simulink model "lab10_2"  (R2016a)
settings: Solver=VariableStepAuto  StartTime=0.0  StopTime=10.0  RelTol=1e-3
libraries: dsparch4 x1, dspsrcs4 x1
settings Model: Creator=Student  LastModifiedBy=Student

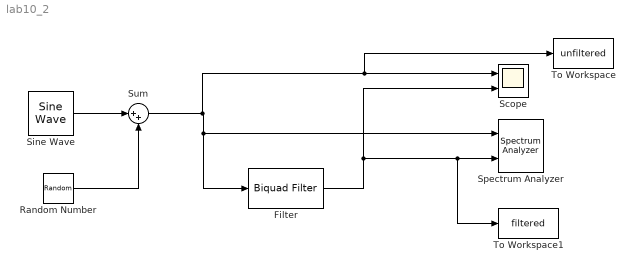
== system lab10_2 ==
  Filter : dsparch4/Biquad Filter  Tag=BlockMethodSubSystem  IIRFiltStruct=Direct form II  CoeffSource=Specify via dialog  BiQuadCoeffs=[1 0 -1 1 -1.9845074082594112 0.99843757775402564;1 0 -1 1 -1.9979478884288948 0.99948076698925981;1 0 -1 1 -1.9814205352744034 0.99532172958549414;1 0 -1 1 -1.9969099740617273 0.9984428591197374;1 0 -1 1 -1.9783555133988198 0.99222061889760815;1 0 -1 1 -1.9958715832818095 0.99740527789565281;1 0 -1 1 -1.9753155281161083 0.98913749900784731;1 0 -1 1 -1.9948322136381669 0.99636752295808573;1 0 -1 1 -1.9723037166687756 0.98607557998158213;1 0 -1 1 -1.9937913609097069 0.99532909405264125;1 0 -1 1 -1.9693231679376586 0.98303802835905307;1 0 -1 1 -1.9927485183051488 0.99428949025058977;1 0 -1 1 -1.9663769224293755 0.98002796699845007;1 0 -1 1 -1.991703175664242 0.99324820918062173;1 0 -1 1 -1.9634679723688206 0.97704847503463499;1 0 -1 1 -1.9906548186594781 0.99220474626846311;1 0 -1 1 -1.960599261888559 0.97410258794139148;1 0 -1 1 -1.9896029280026326 0.99115859399356476;1 0 -1 1 -1.9577736873165876 0.97119329770359009;1 0 -1 1 -1.9885469786503591 0.99010924115306598;1 0 -1 1 -1.9549940975470752 0.96832355308060447;1 0 -1 1 -1.9874864390201967 0.98905617214895281;1 0 -1 1 -1.952263294493517 0.96549625996456945;1 0 -1 1 -1.9864207702131631 0.98799886629153555;1 0 -1 1 -1.9495840336145673 0.96271428182261787;1 0 -1 1 -1.9853494252484865 0.98693679712742777;1 0 -1 1 -1.9469590245001744 0.95998044021271833;1 0 -1 1 -1.9842718483184303 0.98586943179955744;1 0 -1 1 -1.9443909315133903 0.95729751536788832;1 0 -1 1 -1.9831874740635671 0.98479623044188003;1 0 -1 1 -1.9418823744702292 0.95466824683527696;1 0 -1 1 -1.9820957268816377 0.98371664561974226;1 0 -1 1 -1.9394359293472216 0.95209533415765057;1 0 -1 1 -1.980996020276186 0.98263012182637588;1 0 -1 1 -1.9370541290001957 0.94958143758426283;1 0 -1 1 -1.9798877562570185 0.9815360950463432;1 0 -1 1 -1.9347394638708142 0.94712917878769443;1 0 -1 1 -1.9787703248116386 0.98043399240783657;1 0 -1 1 -1.9324943826727332 0.94474114158409206;1 0 -1 1 -1.9776431034517783 0.97932323192445625;1 0 -1 1 -1.9303212930077263 0.94241987260101812;1 0 -1 1 -1.9765054568802456 0.97820322238202739;1 0 -1 1 -1.9282225619104643 0.94016788190406153;1 0 -1 1 -1.9753567367755163 0.97707336335711437;1 0 -1 1 -1.9262005162666878 0.93798764352019337;1 0 -1 1 -1.9741962817452121 0.97593304542962866;1 0 -1 1 -1.9242574430627926 0.93588159582225039;1 0 -1 1 -1.9730234174865544 0.97478165062471533;1 0 -1 1 -1.922395589442883 0.93385214175666553;1 0 -1 1 -1.9718374571739159 0.97361855310047196;1 0 -1 1 -1.9206171624641288 0.9319016487963403;1 0 -1 1 -1.9706377021787449 0.97244312020222756;1 0 -1 1 -1.9189243285601516 0.93003244865059176;1 0 -1 1 -1.9694234431087829 0.97125471384760487;1 0 -1 1 -1.917319212548446 0.92824683655119711;1 0 -1 1 -1.9681939613267141 0.97005269242764869;1 0 -1 1 -1.9158038961485049 0.92654707009800152;1 0 -1 1 -1.9669485309783634 0.96883641323734271;1 0 -1 1 -1.9143804158708309 0.92493536752210992;1 0 -1 1 -1.9656864216668195 0.96760523557834921;1 0 -1 1 -1.9130507601784605 0.92341390527619893;1 0 -1 1 -1.9644069018678416 0.96635852462144056;1 0 -1 1 -1.9118168657299632 0.92198481475696581;1 0 -1 1 -1.9631092432741633 0.96509565622301208;1 0 -1 1 -1.9106806125658913 0.92065017803059168;1 0 -1 1 -1.9617927262041244 0.9638160228186915;1 0 -1 1 -1.9096438180476545 0.91941202237084474;1 0 -1 1 -1.9604566462625255 0.96251904057696724;1 0 -1 1 -1.9087082292948967 0.9182723133557017;1 0 -1 1 -1.9591003225050778 0.96120415805805015;1 0 -1 1 -1.9577231073356889 0.95987086659593657;1 0 -1 1 -1.9078755138892836 0.91723294628854357;1 0 -1 1 -1.9563243983755705 0.95851871261782839;1 0 -1 1 -1.9071472486035819 0.91629573570694711;1 0 -1 1 -1.9549036526803112 0.95714731227285954;1 0 -1 1 -1.9065249057770417 0.91546240258244826;1 0 -1 1 -1.9534604035622678 0.95575636858874891;1 0 -1 1 -1.9060098370778604 0.91473455895150158;1 0 -1 1 -1.951994280334671 0.95434569144367565;1 0 -1 1 -1.9056032543338908 0.91411368964023243;1 0 -1 1 -1.9505050313511418 0.95291522069259427;1 0 -1 1 -1.905306207056062 ...(+1825 chars)Flag=Warning  IC=0  ICnum=0  ICden=0  InputProcessing=Columns as channels (frame based)  denAccumFracLength=30  denProdOutputFracLength=30  secondMemoryFracLength=15  roundingMode=Floor  overflowMode=off  ScaleValues=[0.039462450070613789;0.039462450070613789;0.039421470696737307;0.039421470696737307;0.039380661366385863;0.039380661366385863;0.039340049333478705;0.039340049333478705;0.039299661463220482;0.039299661463220482;0.039259524219459226;0.039259524219459226;0.03921966365291292;0.03921966365291292;0.039180105390243455;0.039180105390243455;0.039140874623955359;0.039140874623955359;0.039101996103095317;0.039101996103095317;0.039063494124727836;0.039063494124727836;0.039025392526161058;0.039025392526161058;0.038987714677896322;0.038987714677896322;0.038950483477274062;0.038950483477274062;0.038913721342788476;0.038913721342788476;0.038877450209042715;0.038877450209042715;0.03884169152231591;0.03884169152231591;0.038806466236713681;0.038806466236713681;0.038771794810872971;0.038771794810872971;0.038737697205192524;0.038737697205192524;0.038704192879560173;0.038704192879560173;0.038671300791548333;0.038671300791548333;0.038639039395049202;0.038639039395049202;0.038607426639321582;0.038607426639321582;0.038576479968421507;0.038576479968421507;0.038546216320989257;0.038546216320989257;0.038516652130365918;0.038516652130365918;0.038487803325012976;0.038487803325012976;0.038459685329209084;0.038459685329209084;0.038432313063998837;0.038432313063998837;0.038405700948368697;0.038405700948368697;0.03837986290062629;0.03837986290062629;0.038354812339959618;0.038354812339959618;0.038330562188153616;0.038330562188153616;0.038307124871442208;0.038307124871442208;0.038284512322474658;0.038284512322474658;0.038262735982375944;0.038262735982375944;0.038241806802881438;0.038241806802881438;0.038221735248527094;0.038221735248527094;0.038202531298877199;0.038202531298877199;0.038184204450772266;0.038184204450772266;0.038166763720580761;0.038166763720580761;0.038150217646438972;0.038150217646438972;0.038134574290464053;0.038134574290464053;0.038119841240926322;0.038119841240926322;0.038106025614367489;0.038106025614367489;0.038093134057652286;0.038093134057652286;0.038081172749941813;0.038081172749941813;0.038070147404577835;0.038070147404577835;0.038060063270867646;0.038060063270867646;0.038050925135760374;0.038050925135760374;0.038042737325406056;0.038042737325406056;0.038035503706589605;0.038035503706589605;0.038029227688032734;0.038029227688032734;0.038023912221557425;0.038023912221557425;0.038019559803105507;0.038019559803105507;0.038016172473609423;0.038016172473609423;0.038013751819710194;0.038013751819710194;0.038012298974319313;0.038012298974319313;0.038011814617021897;1]  optimizeScaleValues=on  ScaleValueMode=Specify via input port (g)  scaleValueFracLength=14  FilterSource=Specify via dialog  FilterObject=BQF
  Random Number : RandomNumber  SampleTime=1/8000
  Scope : Scope  NumInputPorts=2
  Sine Wave : dspsrcs4/Sine Wave  Amplitude=1  Frequency=100  Phase=0  SampleMode=Discrete  OutComplex=Real  CompMethod=Trigonometric fcn  TableSize=Speed  SampleTime=1/8000  SamplesPerFrame=1  ResetState=Restart at time zero  OutputFrames=off  dataType=double  wordLen=16  udDataType=sfix(16)  fracBitsMode=Best precision  numFracBits=15  OutDataTypeStr=double  LastOutDataTypeStr=double
  Spectrum Analyzer : SpectrumAnalyzer  NumInputPorts=2
  Sum : Sum  Inputs=|++
  To Workspace : ToWorkspace  VariableName=unfiltered  SampleTime=-1
      settings: Save2DSignal=2-D array (concatenate along first dimension)
  To Workspace1 : ToWorkspace  VariableName=filtered  SampleTime=-1
      settings: Save2DSignal=2-D array (concatenate along first dimension)
  wires:
  Random Number/1 -> Sum/2
  Sine Wave/1 -> Sum/1
  Sum/1 -> To Workspace/1, Scope/1, Filter/1, Spectrum Analyzer/1
  Filter/1 -> Scope/2, To Workspace1/1, Spectrum Analyzer/2
